simulink model "RW_Model"  (R2024a)
settings: Solver=VariableStepAuto  StartTime=0.0  StopTime=10.0  RelTol=1e-3
values from neighbouring files (symbols this model uses):
  b = 10e-6    (= 1e-05)    [init_SAR_AOCS.m]
  Km = 0.1    [init_SAR_AOCS.m]
  Kt = 0.1    [init_SAR_AOCS.m]
  L = 5.2e-3    (= 0.0052)    [init_SAR_AOCS.m]
  R = 2    [init_SAR_AOCS.m]
  rw_Inertia = 5e-4    (= 0.0005)    [init_SAR_AOCS.m]
  rw_SensorToBody = [0 0.4741 0.4741 -0.9482;                   -0.9999 0.3333 0.3333 0.3333;                    0 -0.8165 0.8165 0 ]    [init_SAR_AOCS.m]
  RW_wmax = 300    [init_SAR_AOCS.m]
  Ts = sim.dt    [init_SAR_AOCS.m]
  w_init = initial.omega    [init_SAR_AOCS.m]
  wRW_init = [0;0;0;0]    [init_SAR_AOCS.m]
libraries: simulink_extras x8, slpidlib x4, simulink x4
settings Model: Creator=hendr  LastModifiedBy=hendr

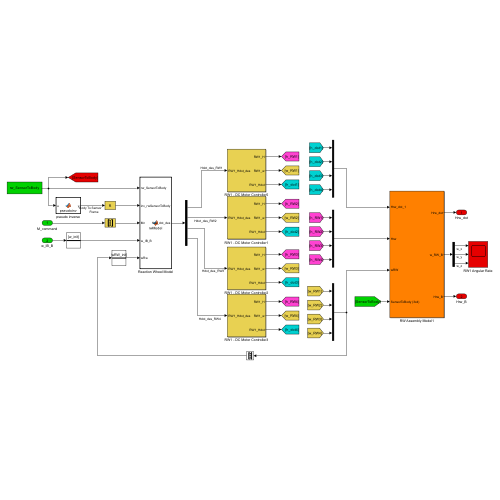
[thumbnail: Simulink's stored preview of the top-level diagram]
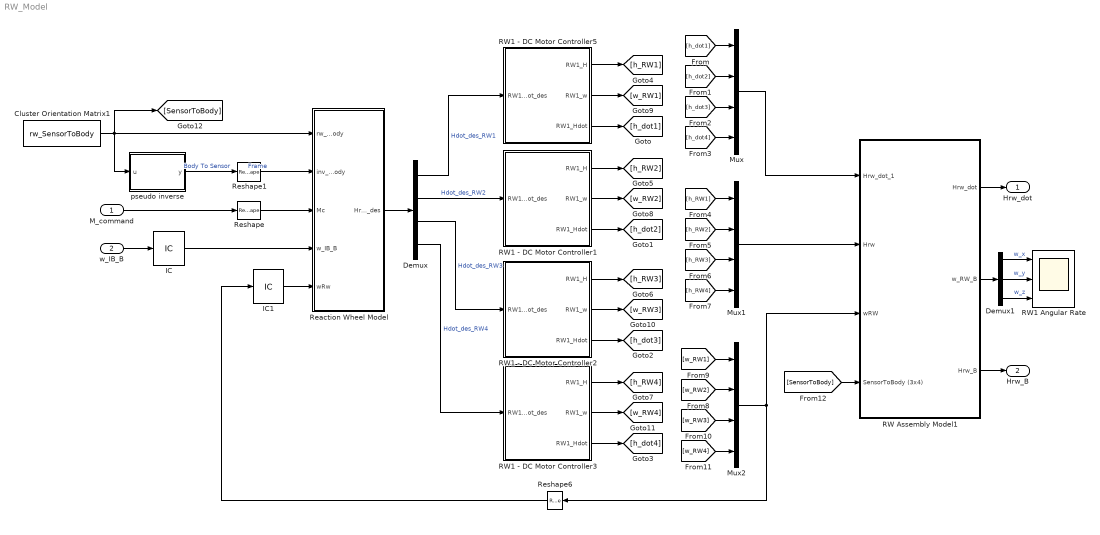
== system RW_Model ==
  "M_command " : Inport
  w_IB_B : Inport  Port=2
  Cluster Orientation Matrix1 : Constant  Value=rw_SensorToBody  VectorParams1D=off  SampleTime=Ts
  Demux : Demux
  Demux1 : Demux  Outputs=3
  IC : InitialCondition  Value=w_init
  IC1 : InitialCondition  Value=wRW_init
  Mux : Mux
  Mux1 : Mux
  Mux2 : Mux
  RW Assembly Model1 : Subsystem
  RW1 - DC Motor Controller1 : Subsystem
  RW1 - DC Motor Controller2 : Subsystem
  RW1 - DC Motor Controller3 : Subsystem
  RW1 - DC Motor Controller5 : Subsystem
  RW1 Angular Rate : Scope  NumInputPorts=3
  Reaction Wheel Model : MATLAB Function  TreatAsAtomicUnit=on
  Reshape : Reshape  OutputDimensionality=Column vector (2-D)
  Reshape1 : Reshape  OutputDimensionality=Customize  OutputDimensions=[4,3]
  Reshape6 : Reshape  OutputDimensionality=Column vector (2-D)
  pseudo inverse : MATLAB Function  TreatAsAtomicUnit=on
  "Hrw_dot " : Outport  VectorParamsAs1DForOutWhenUnconnected=off
  Hrw_B : Outport  Port=2  VectorParamsAs1DForOutWhenUnconnected=off
  wires:
  RW Assembly Model1/3(Hrw_B) -> Hrw_B/1
  Demux/4 -> RW1 - DC Motor Controller3/1(RW1_Hdot_des)  "Hdot_des_RW4"
  IC1/1 -> Reaction Wheel Model/5(wRw)
  Mux2/1 -> Reshape6/1, RW Assembly Model1/3(wRW)
  Reshape6/1 -> IC1/1
  RW1 - DC Motor Controller3/2(RW1_w) -> [w_RW4]
  RW1 - DC Motor Controller2/1(RW1_H) -> [h_RW3]
  RW1 - DC Motor Controller5/2(RW1_w) -> [w_RW1]
  [w_RW3] -> Mux2/3
  RW Assembly Model1/2(w_RW_B) -> Demux1/1
  RW1 - DC Motor Controller5/3(RW1_Hdot) -> [h_dot1]
  RW1 - DC Motor Controller3/3(RW1_Hdot) -> [h_dot4]
  RW1 - DC Motor Controller2/2(RW1_w) -> [w_RW3]
  RW1 - DC Motor Controller1/3(RW1_Hdot) -> [h_dot2]
  [h_dot3] -> Mux/3
  Demux/1 -> RW1 - DC Motor Controller5/1(RW1_Hdot_des)  "Hdot_des_RW1"
  RW1 - DC Motor Controller5/1(RW1_H) -> [h_RW1]
  RW1 - DC Motor Controller1/2(RW1_w) -> [w_RW2]
  RW1 - DC Motor Controller1/1(RW1_H) -> [h_RW2]
  RW1 - DC Motor Controller3/1(RW1_H) -> [h_RW4]
  RW1 - DC Motor Controller2/3(RW1_Hdot) -> [h_dot3]
  [h_RW3] -> Mux1/3
  Reshape1/1 -> Reaction Wheel Model/2(inv_rwSensorToBody)
  [SensorToBody] -> RW Assembly Model1/4(SensorToBody (3x4))
  "M_command "/1 -> Reshape/1
  Mux/1 -> RW Assembly Model1/1(Hrw_dot_1)
  Reshape/1 -> Reaction Wheel Model/3(Mc)
  pseudo inverse/1(y) -> Reshape1/1  "Body To Sensor         Frame"
  w_IB_B/1 -> IC/1
  Demux/2 -> RW1 - DC Motor Controller1/1(RW1_Hdot_des)  "Hdot_des_RW2"
  [h_RW2] -> Mux1/2
  RW Assembly Model1/1(Hrw_dot) -> "Hrw_dot "/1
  IC/1 -> Reaction Wheel Model/4(w_IB_B)
  [h_RW4] -> Mux1/4
  Demux1/3 -> RW1 Angular Rate/3  "w_z"
  [w_RW2] -> Mux2/2
  [h_RW1] -> Mux1/1
  [h_dot2] -> Mux/2
  Reaction Wheel Model/1(Hrw_dot_des) -> Demux/1
  [w_RW1] -> Mux2/1
  Demux/3 -> RW1 - DC Motor Controller2/1(RW1_Hdot_des)  "Hdot_des_RW3"
  Mux1/1 -> RW Assembly Model1/2(Hrw)
  [h_dot4] -> Mux/4
  [w_RW4] -> Mux2/4
  Cluster Orientation Matrix1/1 -> pseudo inverse/1(u), [SensorToBody], Reaction Wheel Model/1(rw_SensorToBody)
  Demux1/1 -> RW1 Angular Rate/1  "w_x"
  [h_dot1] -> Mux/1
  Demux1/2 -> RW1 Angular Rate/2  "w_y"

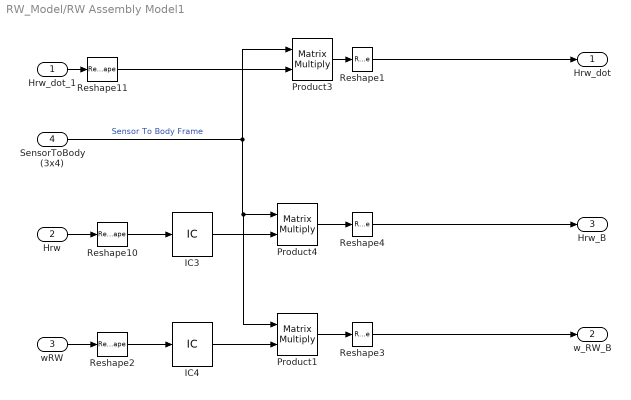
== system RW_Model/RW Assembly Model1 ==
  Hrw_dot_1 : Inport
  Hrw : Inport  Port=2
  wRW : Inport  Port=3
  SensorToBody (3x4) : Inport  Port=4
  IC3 : InitialCondition  Value=[wRW_init(1,1)*rw_Inertia; wRW_init(2,1)*rw_Inertia; wRW_init(3,1)*rw_Inertia;wRW_init(4,1)*rw_Inertia]
  IC4 : InitialCondition  Value=wRW_init
  Product1 : Product  Inputs=**  Multiplication=Matrix(*)  RndMeth=Zero
  Product3 : Product  Inputs=**  Multiplication=Matrix(*)  RndMeth=Zero
  Product4 : Product  Inputs=**  Multiplication=Matrix(*)  RndMeth=Zero
  Reshape{1..4,10..11} (6 alike) : Reshape  OutputDimensionality=Column vector (2-D)
  Hrw_dot : Outport  VectorParamsAs1DForOutWhenUnconnected=off
  w_RW_B : Outport  Port=2  VectorParamsAs1DForOutWhenUnconnected=off
  Hrw_B : Outport  Port=3  VectorParamsAs1DForOutWhenUnconnected=off
  wires:
  SensorToBody (3x4)/1 -> Product3/1, Product1/1, Product4/1  "Sensor To Body Frame"
  Product4/1 -> Reshape4/1
  Reshape1/1 -> Hrw_dot/1
  Reshape4/1 -> Hrw_B/1
  IC3/1 -> Product4/2
  IC4/1 -> Product1/2
  Product1/1 -> Reshape3/1
  Hrw/1 -> Reshape10/1
  Reshape10/1 -> IC3/1
  Reshape2/1 -> IC4/1
  wRW/1 -> Reshape2/1
  Reshape3/1 -> w_RW_B/1
  Reshape11/1 -> Product3/2
  Hrw_dot_1/1 -> Reshape11/1
  Product3/1 -> Reshape1/1

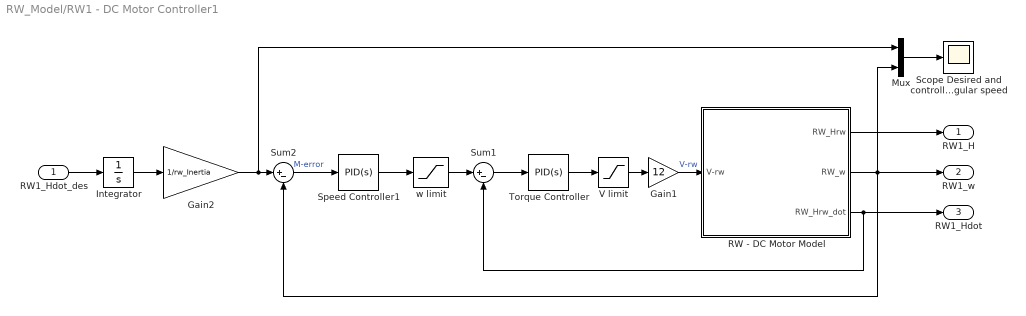
== system RW_Model/RW1 - DC Motor Controller1 ==
  RW1_Hdot_des : Inport
  Gain1 : Gain  Gain=12
  Gain2 : Gain  Gain=1/rw_Inertia
  Integrator : Integrator
  Mux : Mux  Inputs=2
  RW - DC Motor Model : Subsystem
  "Scope Desired and controlled RW-angular speed " : Scope
  Speed Controller1 : slpidlib/PID Controller  Controller=PID  Form=Parallel  TimeDomain=Continuous-time  UseExternalTs=off  SampleTime=0.01  IntegratorMethod=Forward Euler  FilterMethod=Forward Euler  ControllerParametersSource=internal  P=9.56052273582853  I=13.4366327144231  UseKiTs=off  D=1.16248121318414  UseExternalDerivativeSource=off  N=2668.95305381072  UseFilter=on  TunerSelectOption=Transfer Function Based (PID Tuner App)  InitialConditionSource=internal  InitialConditionForIntegrator=0  InitialConditionForFilter=0  DifferentiatorICPrevScaledInput=0  ExternalReset=none  TrackingMode=off  Kt=1  LimitOutput=off  SatLimitsSource=internal  UpperSaturationLimit=inf  LowerSaturationLimit=-inf  LinearizeAsGain=on  AntiWindupMode=none  Kb=1  LimitIntegrator=off  UpperIntegratorSaturationLimit=inf  LowerIntegratorSaturationLimit=-inf  POutMin=[]  POutMax=[]  IOutMin=[]  IOutMax=[]  DOutMin=[]  DOutMax=[]  NOutMin=[]  NOutMax=[]  SumOutMin=[]  SumOutMax=[]  SaturationOutMin=[]  SaturationOutMax=[]  PParamMin=[]  PParamMax=[]  IParamMin=[]  IParamMax=[]  DParamMin=[]  DParamMax=[]  NParamMin=[]  NParamMax=[]  KbParamMin=[]  KbParamMax=[]  KtParamMin=[]  KtParamMax=[]  KbOutMin=[]  KbOutMax=[]  KtOutMin=[]  KtOutMax=[]  IntegratorOutMin=[]  IntegratorOutMax=[]  FilterOutMin=[]  FilterOutMax=[]  SumI1OutMin=[]  SumI1OutMax=[]  SumI2OutMin=[]  SumI2OutMax=[]  SumI3OutMin=[]  SumI3OutMax=[]  SumI4OutMin=[]  SumI4OutMax=[]  SumDOutMin=[]  SumDOutMax=[]  DifferentiatorOutMin=[]  DifferentiatorOutMax=[]  FilterDiffOutCoefMin=[]  FilterDiffOutCoefMax=[]  ReciprocalOutMin=[]  ReciprocalOutMax=[]  SumDenOutMin=[]  SumDenOutMax=[]  SumNumOutMin=[]  SumNumOutMax=[]  DivideOutMin=[]  DivideOutMax=[]  UdiffTsProdOutMin=[]  UdiffTsProdOutMax=[]  NTsProdOutMin=[]  NTsProdOutMax=[]  UintegralTsProdOutMin=[]  UintegralTsProdOutMax=[]  UngainTsProdOutMin=[]  UngainTsProdOutMax=[]  ClampingZeroOutDataTypeStr=Inherit: Inherit via back propagation  ClampingZeroOutMin=[]  ClampingZeroOutMax=[]  FilterDenConstantOutDataTypeStr=Inherit: Inherit via back propagation  FilterDenConstantOutMin=[]  FilterDenConstantOutMax=[]  PCopyOutDataTypeStr=Inherit: Inherit via back propagation  PCopyOutMin=[]  PCopyOutMax=[]  NCopyOutDataTypeStr=Inherit: Inherit via back propagation  NCopyOutMin=[]  NCopyOutMax=[]  IntegratorContinuousStateAttributes=''  IntegratorStateMustResolveToSignalObject=off  IntegratorRTWStateStorageClass=Auto  FilterContinuousStateAttributes=''  FilterStateMustResolveToSignalObject=off  FilterRTWStateStorageClass=Auto  ParallelPVariant=InternalParameters  IdealPVariant=Disabled  IVariant=InternalParameters  DVariant=InternalParameters  IntegratorVariant=Continuous  SatVariant=Disabled  AWVariant=Passthrough  PCopyVariant=Disabled  TRVariant=Disabled  FdbkBlocksVariant=Forward  IdealPFdbkVariant=Disabled  SatFdbkVariant=Disabled  DerivativeFilterVariant=ContFilter  NVariant=InternalParameters  NCopyVariant=Disabled  FilterICVariant=InternalICsFilter  IntegratorICVariant=InternalICs  ExternalResetVariant=Disabled  TRSumVariant=Passthrough  SumFdbkVariant=Disabled  SumVariant=Sum_PID  TsampFilterVariant=InternalTs  TsampNgainVariant=Passthrough  TsampIntegralVariant=Disabled_SignalSpec  ExternalSaturationOutDataTypeStr=Inherit: Same as second input  DerivativeSourceVariant=ErrorSignal
  Sum1 : Sum  Inputs=|+-
  Sum2 : Sum  Inputs=|+-
  Torque Controller : slpidlib/PID Controller  Controller=PID  Form=Parallel  TimeDomain=Continuous-time  UseExternalTs=off  SampleTime=0.01  IntegratorMethod=Forward Euler  FilterMethod=Forward Euler  ControllerParametersSource=internal  P=2.50374683332827e-05  I=0.022215359014968  UseKiTs=off  D=0  UseExternalDerivativeSource=off  N=100  UseFilter=on  TunerSelectOption=Transfer Function Based (PID Tuner App)  InitialConditionSource=internal  InitialConditionForIntegrator=0  InitialConditionForFilter=0  DifferentiatorICPrevScaledInput=0  ExternalReset=none  TrackingMode=off  Kt=1  LimitOutput=off  SatLimitsSource=internal  UpperSaturationLimit=inf  LowerSaturationLimit=-inf  LinearizeAsGain=on  AntiWindupMode=none  Kb=1  LimitIntegrator=off  UpperIntegratorSaturationLimit=inf  LowerIntegratorSaturationLimit=-inf  POutMin=[]  POutMax=[]  IOutMin=[]  IOutMax=[]  DOutMin=[]  DOutMax=[]  NOutMin=[]  NOutMax=[]  SumOutMin=[]  SumOutMax=[]  SaturationOutMin=[]  SaturationOutMax=[]  PParamMin=[]  PParamMax=[]  IParamMin=[]  IParamMax=[]  DParamMin=[]  DParamMax=[]  NParamMin=[]  NParamMax=[]  KbParamMin=[]  KbParamMax=[]  KtParamMin=[]  KtParamMax=[]  KbOutMin=[]  KbOutMax=[]  KtOutMin=[]  KtOutMax=[]  IntegratorOutMin=[]  IntegratorOutMax=[]  FilterOutMin=[]  FilterOutMax=[]  SumI1OutMin=[]  SumI1OutMax=[]  SumI2OutMin=[]  SumI2OutMax=[]  SumI3OutMin=[]  SumI3OutMax=[]  SumI4OutMin=[]  SumI4OutMax=[]  SumDOutMin=[]  SumDOutMax=[]  DifferentiatorOutMin=[]  DifferentiatorOutMax=[]  FilterDiffOutCoefMin=[]  FilterDiffOutCoefMax=[]  ReciprocalOutMin=[]  ReciprocalOutMax=[]  SumDenOutMin=[]  SumDenOutMax=[]  SumNumOutMin=[]  SumNumOutMax=[]  DivideOutMin=[]  DivideOutMax=[]  UdiffTsProdOutMin=[]  UdiffTsProdOutMax=[]  NTsProdOutMin=[]  NTsProdOutMax=[]  UintegralTsProdOutMin=[]  UintegralTsProdOutMax=[]  UngainTsProdOutMin=[]  UngainTsProdOutMax=[]  ClampingZeroOutDataTypeStr=Inherit: Inherit via back propagation  ClampingZeroOutMin=[]  ClampingZeroOutMax=[]  FilterDenConstantOutDataTypeStr=Inherit: Inherit via back propagation  FilterDenConstantOutMin=[]  FilterDenConstantOutMax=[]  PCopyOutDataTypeStr=Inherit: Inherit via back propagation  PCopyOutMin=[]  PCopyOutMax=[]  NCopyOutDataTypeStr=Inherit: Inherit via back propagation  NCopyOutMin=[]  NCopyOutMax=[]  IntegratorContinuousStateAttributes=''  IntegratorStateMustResolveToSignalObject=off  IntegratorRTWStateStorageClass=Auto  FilterContinuousStateAttributes=''  FilterStateMustResolveToSignalObject=off  FilterRTWStateStorageClass=Auto  ParallelPVariant=InternalParameters  IdealPVariant=Disabled  IVariant=InternalParameters  DVariant=InternalParameters  IntegratorVariant=Continuous  SatVariant=Disabled  AWVariant=Passthrough  PCopyVariant=Disabled  TRVariant=Disabled  FdbkBlocksVariant=Forward  IdealPFdbkVariant=Disabled  SatFdbkVariant=Disabled  DerivativeFilterVariant=ContFilter  NVariant=InternalParameters  NCopyVariant=Disabled  FilterICVariant=InternalICsFilter  IntegratorICVariant=InternalICs  ExternalResetVariant=Disabled  TRSumVariant=Passthrough  SumFdbkVariant=Disabled  SumVariant=Sum_PID  TsampFilterVariant=InternalTs  TsampNgainVariant=Passthrough  TsampIntegralVariant=Disabled_SignalSpec  ExternalSaturationOutDataTypeStr=Inherit: Same as second input  DerivativeSourceVariant=ErrorSignal
  V limit : Saturate  UpperLimit=20  LowerLimit=-20
  w limit : Saturate  UpperLimit=RW_wmax  LowerLimit=-RW_wmax
  RW1_H : Outport  VectorParamsAs1DForOutWhenUnconnected=off
  RW1_w : Outport  Port=2  VectorParamsAs1DForOutWhenUnconnected=off
  RW1_Hdot : Outport  Port=3  VectorParamsAs1DForOutWhenUnconnected=off
  wires:
  Torque Controller/1 -> V limit/1
  RW - DC Motor Model/3(RW_Hrw_dot) -> RW1_Hdot/1, Sum1/2
  Mux/1 -> "Scope Desired and controlled RW-angular speed "/1
  V limit/1 -> Gain1/1
  Gain1/1 -> RW - DC Motor Model/1(V-rw)  "V-rw"
  RW - DC Motor Model/2(RW_w) -> RW1_w/1, Sum2/2, Mux/2
  Sum1/1 -> Torque Controller/1
  RW - DC Motor Model/1(RW_Hrw) -> RW1_H/1
  Speed Controller1/1 -> w limit/1
  w limit/1 -> Sum1/1
  Sum2/1 -> Speed Controller1/1  "M-error"
  Integrator/1 -> Gain2/1
  RW1_Hdot_des/1 -> Integrator/1
  Gain2/1 -> Mux/1, Sum2/1

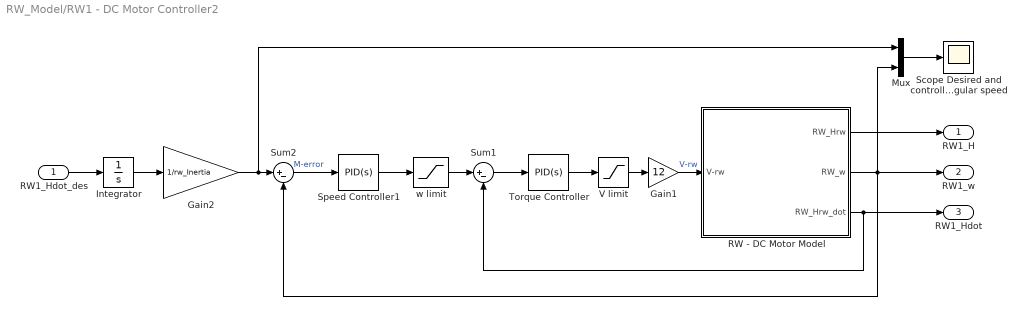
== system RW_Model/RW1 - DC Motor Controller2 ==
  RW1_Hdot_des : Inport
  Gain1 : Gain  Gain=12
  Gain2 : Gain  Gain=1/rw_Inertia
  Integrator : Integrator
  Mux : Mux  Inputs=2
  RW - DC Motor Model : Subsystem
  "Scope Desired and controlled RW-angular speed " : Scope
  Speed Controller1 : simulink/Continuous/PID Controller  Controller=PID  Form=Parallel  TimeDomain=Continuous-time  SampleTime=0.01  IntegratorMethod=Forward Euler  FilterMethod=Forward Euler  ControllerParametersSource=internal  P=9.56052273582853  I=13.4366327144231  D=1.16248121318414  UseFilter=on  N=2668.95305381072  TunerSelectOption=Transfer Function Based (PID Tuner App)  InitialConditionSource=internal  InitialConditionForIntegrator=0  InitialConditionForFilter=0  DifferentiatorICPrevScaledInput=0  ExternalReset=none  TrackingMode=off  Kt=1  LimitOutput=off  UpperSaturationLimit=inf  LowerSaturationLimit=-inf  LinearizeAsGain=on  AntiWindupMode=none  Kb=1  POutMin=[]  POutMax=[]  IOutMin=[]  IOutMax=[]  DOutMin=[]  DOutMax=[]  NOutMin=[]  NOutMax=[]  SumOutMin=[]  SumOutMax=[]  SaturationOutMin=[]  SaturationOutMax=[]  PParamMin=[]  PParamMax=[]  IParamMin=[]  IParamMax=[]  DParamMin=[]  DParamMax=[]  NParamMin=[]  NParamMax=[]  KbParamMin=[]  KbParamMax=[]  KtParamMin=[]  KtParamMax=[]  KbOutMin=[]  KbOutMax=[]  KtOutMin=[]  KtOutMax=[]  IntegratorOutMin=[]  IntegratorOutMax=[]  FilterOutMin=[]  FilterOutMax=[]  SumI1OutMin=[]  SumI1OutMax=[]  SumI2OutMin=[]  SumI2OutMax=[]  SumI3OutMin=[]  SumI3OutMax=[]  SumI4OutMin=[]  SumI4OutMax=[]  SumDOutMin=[]  SumDOutMax=[]  DifferentiatorOutMin=[]  DifferentiatorOutMax=[]  FilterDiffOutCoefMin=[]  FilterDiffOutCoefMax=[]  ReciprocalOutMin=[]  ReciprocalOutMax=[]  SumDenOutMin=[]  SumDenOutMax=[]  SumNumOutMin=[]  SumNumOutMax=[]  DivideOutMin=[]  DivideOutMax=[]  IntegratorContinuousStateAttributes=''  IntegratorStateMustResolveToSignalObject=off  IntegratorRTWStateStorageClass=Auto  FilterContinuousStateAttributes=''  FilterStateMustResolveToSignalObject=off  FilterRTWStateStorageClass=Auto  ParallelPVariant=InternalParameters  IdealPVariant=Disabled  IVariant=InternalParameters  DVariant=InternalParameters  IntegratorVariant=Continuous  SatVariant=Disabled  AWVariant=Passthrough  PCopyVariant=Disabled  TRVariant=Disabled  FdbkBlocksVariant=Forward  IdealPFdbkVariant=Disabled  SatFdbkVariant=Disabled  DerivativeFilterVariant=ContFilter  NVariant=InternalParameters  NCopyVariant=Disabled  FilterICVariant=InternalICsFilter  IntegratorICVariant=InternalICs  ExternalResetVariant=Disabled  TRSumVariant=Passthrough  SumFdbkVariant=Disabled  SumVariant=Sum_PID
  Sum1 : Sum  Inputs=|+-
  Sum2 : Sum  Inputs=|+-
  Torque Controller : simulink/Continuous/PID Controller  Controller=PID  Form=Parallel  TimeDomain=Continuous-time  SampleTime=0.01  IntegratorMethod=Forward Euler  FilterMethod=Forward Euler  ControllerParametersSource=internal  P=2.50374683332827e-05  I=0.022215359014968  D=0  UseFilter=on  N=100  TunerSelectOption=Transfer Function Based (PID Tuner App)  InitialConditionSource=internal  InitialConditionForIntegrator=0  InitialConditionForFilter=0  DifferentiatorICPrevScaledInput=0  ExternalReset=none  TrackingMode=off  Kt=1  LimitOutput=off  UpperSaturationLimit=inf  LowerSaturationLimit=-inf  LinearizeAsGain=on  AntiWindupMode=none  Kb=1  POutMin=[]  POutMax=[]  IOutMin=[]  IOutMax=[]  DOutMin=[]  DOutMax=[]  NOutMin=[]  NOutMax=[]  SumOutMin=[]  SumOutMax=[]  SaturationOutMin=[]  SaturationOutMax=[]  PParamMin=[]  PParamMax=[]  IParamMin=[]  IParamMax=[]  DParamMin=[]  DParamMax=[]  NParamMin=[]  NParamMax=[]  KbParamMin=[]  KbParamMax=[]  KtParamMin=[]  KtParamMax=[]  KbOutMin=[]  KbOutMax=[]  KtOutMin=[]  KtOutMax=[]  IntegratorOutMin=[]  IntegratorOutMax=[]  FilterOutMin=[]  FilterOutMax=[]  SumI1OutMin=[]  SumI1OutMax=[]  SumI2OutMin=[]  SumI2OutMax=[]  SumI3OutMin=[]  SumI3OutMax=[]  SumI4OutMin=[]  SumI4OutMax=[]  SumDOutMin=[]  SumDOutMax=[]  DifferentiatorOutMin=[]  DifferentiatorOutMax=[]  FilterDiffOutCoefMin=[]  FilterDiffOutCoefMax=[]  ReciprocalOutMin=[]  ReciprocalOutMax=[]  SumDenOutMin=[]  SumDenOutMax=[]  SumNumOutMin=[]  SumNumOutMax=[]  DivideOutMin=[]  DivideOutMax=[]  IntegratorContinuousStateAttributes=''  IntegratorStateMustResolveToSignalObject=off  IntegratorRTWStateStorageClass=Auto  FilterContinuousStateAttributes=''  FilterStateMustResolveToSignalObject=off  FilterRTWStateStorageClass=Auto  ParallelPVariant=InternalParameters  IdealPVariant=Disabled  IVariant=InternalParameters  DVariant=InternalParameters  IntegratorVariant=Continuous  SatVariant=Disabled  AWVariant=Passthrough  PCopyVariant=Disabled  TRVariant=Disabled  FdbkBlocksVariant=Forward  IdealPFdbkVariant=Disabled  SatFdbkVariant=Disabled  DerivativeFilterVariant=ContFilter  NVariant=InternalParameters  NCopyVariant=Disabled  FilterICVariant=InternalICsFilter  IntegratorICVariant=InternalICs  ExternalResetVariant=Disabled  TRSumVariant=Passthrough  SumFdbkVariant=Disabled  SumVariant=Sum_PID
  V limit : Saturate  UpperLimit=20  LowerLimit=-20
  w limit : Saturate  UpperLimit=RW_wmax  LowerLimit=-RW_wmax
  RW1_H : Outport  VectorParamsAs1DForOutWhenUnconnected=off
  RW1_w : Outport  Port=2  VectorParamsAs1DForOutWhenUnconnected=off
  RW1_Hdot : Outport  Port=3  VectorParamsAs1DForOutWhenUnconnected=off
  wires:
  Torque Controller/1 -> V limit/1
  RW - DC Motor Model/3(RW_Hrw_dot) -> RW1_Hdot/1, Sum1/2
  Mux/1 -> "Scope Desired and controlled RW-angular speed "/1
  V limit/1 -> Gain1/1
  Gain1/1 -> RW - DC Motor Model/1(V-rw)  "V-rw"
  RW - DC Motor Model/2(RW_w) -> RW1_w/1, Sum2/2, Mux/2
  Sum1/1 -> Torque Controller/1
  RW - DC Motor Model/1(RW_Hrw) -> RW1_H/1
  Speed Controller1/1 -> w limit/1
  w limit/1 -> Sum1/1
  Sum2/1 -> Speed Controller1/1  "M-error"
  Integrator/1 -> Gain2/1
  RW1_Hdot_des/1 -> Integrator/1
  Gain2/1 -> Mux/1, Sum2/1

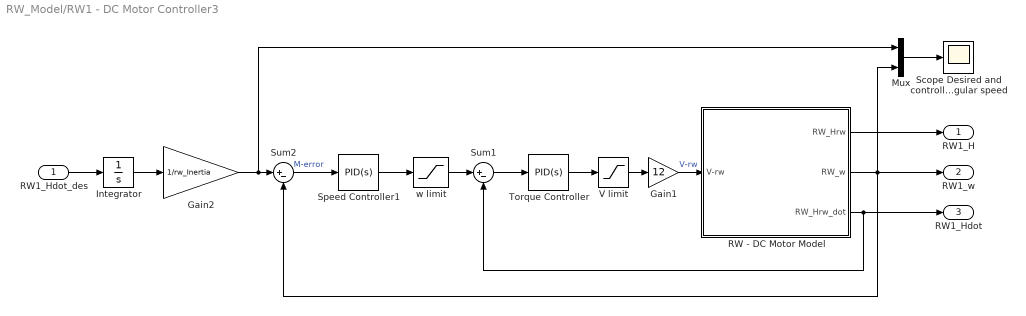
== system RW_Model/RW1 - DC Motor Controller3 ==
  RW1_Hdot_des : Inport
  Gain1 : Gain  Gain=12
  Gain2 : Gain  Gain=1/rw_Inertia
  Integrator : Integrator
  Mux : Mux  Inputs=2
  RW - DC Motor Model : Subsystem
  "Scope Desired and controlled RW-angular speed " : Scope
  Speed Controller1 : simulink/Continuous/PID Controller  Controller=PID  Form=Parallel  TimeDomain=Continuous-time  SampleTime=0.01  IntegratorMethod=Forward Euler  FilterMethod=Forward Euler  ControllerParametersSource=internal  P=9.56052273582853  I=13.4366327144231  D=1.16248121318414  UseFilter=on  N=2668.95305381072  TunerSelectOption=Transfer Function Based (PID Tuner App)  InitialConditionSource=internal  InitialConditionForIntegrator=0  InitialConditionForFilter=0  DifferentiatorICPrevScaledInput=0  ExternalReset=none  TrackingMode=off  Kt=1  LimitOutput=off  UpperSaturationLimit=inf  LowerSaturationLimit=-inf  LinearizeAsGain=on  AntiWindupMode=none  Kb=1  POutMin=[]  POutMax=[]  IOutMin=[]  IOutMax=[]  DOutMin=[]  DOutMax=[]  NOutMin=[]  NOutMax=[]  SumOutMin=[]  SumOutMax=[]  SaturationOutMin=[]  SaturationOutMax=[]  PParamMin=[]  PParamMax=[]  IParamMin=[]  IParamMax=[]  DParamMin=[]  DParamMax=[]  NParamMin=[]  NParamMax=[]  KbParamMin=[]  KbParamMax=[]  KtParamMin=[]  KtParamMax=[]  KbOutMin=[]  KbOutMax=[]  KtOutMin=[]  KtOutMax=[]  IntegratorOutMin=[]  IntegratorOutMax=[]  FilterOutMin=[]  FilterOutMax=[]  SumI1OutMin=[]  SumI1OutMax=[]  SumI2OutMin=[]  SumI2OutMax=[]  SumI3OutMin=[]  SumI3OutMax=[]  SumI4OutMin=[]  SumI4OutMax=[]  SumDOutMin=[]  SumDOutMax=[]  DifferentiatorOutMin=[]  DifferentiatorOutMax=[]  FilterDiffOutCoefMin=[]  FilterDiffOutCoefMax=[]  ReciprocalOutMin=[]  ReciprocalOutMax=[]  SumDenOutMin=[]  SumDenOutMax=[]  SumNumOutMin=[]  SumNumOutMax=[]  DivideOutMin=[]  DivideOutMax=[]  IntegratorContinuousStateAttributes=''  IntegratorStateMustResolveToSignalObject=off  IntegratorRTWStateStorageClass=Auto  FilterContinuousStateAttributes=''  FilterStateMustResolveToSignalObject=off  FilterRTWStateStorageClass=Auto  ParallelPVariant=InternalParameters  IdealPVariant=Disabled  IVariant=InternalParameters  DVariant=InternalParameters  IntegratorVariant=Continuous  SatVariant=Disabled  AWVariant=Passthrough  PCopyVariant=Disabled  TRVariant=Disabled  FdbkBlocksVariant=Forward  IdealPFdbkVariant=Disabled  SatFdbkVariant=Disabled  DerivativeFilterVariant=ContFilter  NVariant=InternalParameters  NCopyVariant=Disabled  FilterICVariant=InternalICsFilter  IntegratorICVariant=InternalICs  ExternalResetVariant=Disabled  TRSumVariant=Passthrough  SumFdbkVariant=Disabled  SumVariant=Sum_PID
  Sum1 : Sum  Inputs=|+-
  Sum2 : Sum  Inputs=|+-
  Torque Controller : simulink/Continuous/PID Controller  Controller=PID  Form=Parallel  TimeDomain=Continuous-time  SampleTime=0.01  IntegratorMethod=Forward Euler  FilterMethod=Forward Euler  ControllerParametersSource=internal  P=2.50374683332827e-05  I=0.022215359014968  D=0  UseFilter=on  N=100  TunerSelectOption=Transfer Function Based (PID Tuner App)  InitialConditionSource=internal  InitialConditionForIntegrator=0  InitialConditionForFilter=0  DifferentiatorICPrevScaledInput=0  ExternalReset=none  TrackingMode=off  Kt=1  LimitOutput=off  UpperSaturationLimit=inf  LowerSaturationLimit=-inf  LinearizeAsGain=on  AntiWindupMode=none  Kb=1  POutMin=[]  POutMax=[]  IOutMin=[]  IOutMax=[]  DOutMin=[]  DOutMax=[]  NOutMin=[]  NOutMax=[]  SumOutMin=[]  SumOutMax=[]  SaturationOutMin=[]  SaturationOutMax=[]  PParamMin=[]  PParamMax=[]  IParamMin=[]  IParamMax=[]  DParamMin=[]  DParamMax=[]  NParamMin=[]  NParamMax=[]  KbParamMin=[]  KbParamMax=[]  KtParamMin=[]  KtParamMax=[]  KbOutMin=[]  KbOutMax=[]  KtOutMin=[]  KtOutMax=[]  IntegratorOutMin=[]  IntegratorOutMax=[]  FilterOutMin=[]  FilterOutMax=[]  SumI1OutMin=[]  SumI1OutMax=[]  SumI2OutMin=[]  SumI2OutMax=[]  SumI3OutMin=[]  SumI3OutMax=[]  SumI4OutMin=[]  SumI4OutMax=[]  SumDOutMin=[]  SumDOutMax=[]  DifferentiatorOutMin=[]  DifferentiatorOutMax=[]  FilterDiffOutCoefMin=[]  FilterDiffOutCoefMax=[]  ReciprocalOutMin=[]  ReciprocalOutMax=[]  SumDenOutMin=[]  SumDenOutMax=[]  SumNumOutMin=[]  SumNumOutMax=[]  DivideOutMin=[]  DivideOutMax=[]  IntegratorContinuousStateAttributes=''  IntegratorStateMustResolveToSignalObject=off  IntegratorRTWStateStorageClass=Auto  FilterContinuousStateAttributes=''  FilterStateMustResolveToSignalObject=off  FilterRTWStateStorageClass=Auto  ParallelPVariant=InternalParameters  IdealPVariant=Disabled  IVariant=InternalParameters  DVariant=InternalParameters  IntegratorVariant=Continuous  SatVariant=Disabled  AWVariant=Passthrough  PCopyVariant=Disabled  TRVariant=Disabled  FdbkBlocksVariant=Forward  IdealPFdbkVariant=Disabled  SatFdbkVariant=Disabled  DerivativeFilterVariant=ContFilter  NVariant=InternalParameters  NCopyVariant=Disabled  FilterICVariant=InternalICsFilter  IntegratorICVariant=InternalICs  ExternalResetVariant=Disabled  TRSumVariant=Passthrough  SumFdbkVariant=Disabled  SumVariant=Sum_PID
  V limit : Saturate  UpperLimit=20  LowerLimit=-20
  w limit : Saturate  UpperLimit=RW_wmax  LowerLimit=-RW_wmax
  RW1_H : Outport  VectorParamsAs1DForOutWhenUnconnected=off
  RW1_w : Outport  Port=2  VectorParamsAs1DForOutWhenUnconnected=off
  RW1_Hdot : Outport  Port=3  VectorParamsAs1DForOutWhenUnconnected=off
  wires:
  Torque Controller/1 -> V limit/1
  RW - DC Motor Model/3(RW_Hrw_dot) -> RW1_Hdot/1, Sum1/2
  Mux/1 -> "Scope Desired and controlled RW-angular speed "/1
  V limit/1 -> Gain1/1
  Gain1/1 -> RW - DC Motor Model/1(V-rw)  "V-rw"
  RW - DC Motor Model/2(RW_w) -> RW1_w/1, Sum2/2, Mux/2
  Sum1/1 -> Torque Controller/1
  RW - DC Motor Model/1(RW_Hrw) -> RW1_H/1
  Speed Controller1/1 -> w limit/1
  w limit/1 -> Sum1/1
  Sum2/1 -> Speed Controller1/1  "M-error"
  Integrator/1 -> Gain2/1
  RW1_Hdot_des/1 -> Integrator/1
  Gain2/1 -> Mux/1, Sum2/1

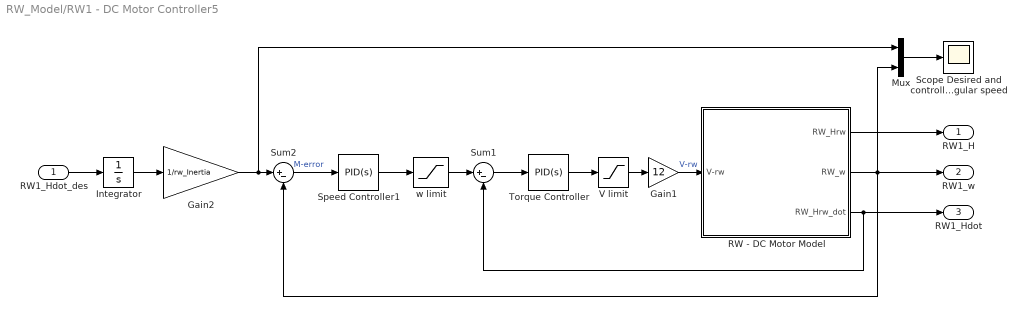
== system RW_Model/RW1 - DC Motor Controller5 ==
  RW1_Hdot_des : Inport
  Gain1 : Gain  Gain=12
  Gain2 : Gain  Gain=1/rw_Inertia
  Integrator : Integrator
  Mux : Mux  Inputs=2
  RW - DC Motor Model : Subsystem
  "Scope Desired and controlled RW-angular speed " : Scope
  Speed Controller1 : slpidlib/PID Controller  Controller=PID  Form=Parallel  TimeDomain=Continuous-time  UseExternalTs=off  SampleTime=0.01  IntegratorMethod=Forward Euler  FilterMethod=Forward Euler  ControllerParametersSource=internal  P=9.56052273582853  I=13.4366327144231  UseKiTs=off  D=1.16248121318414  UseExternalDerivativeSource=off  N=2668.95305381072  UseFilter=on  TunerSelectOption=Transfer Function Based (PID Tuner App)  InitialConditionSource=internal  InitialConditionForIntegrator=0  InitialConditionForFilter=0  DifferentiatorICPrevScaledInput=0  ExternalReset=none  TrackingMode=off  Kt=1  LimitOutput=off  SatLimitsSource=internal  UpperSaturationLimit=inf  LowerSaturationLimit=-inf  LinearizeAsGain=on  AntiWindupMode=none  Kb=1  LimitIntegrator=off  UpperIntegratorSaturationLimit=inf  LowerIntegratorSaturationLimit=-inf  POutMin=[]  POutMax=[]  IOutMin=[]  IOutMax=[]  DOutMin=[]  DOutMax=[]  NOutMin=[]  NOutMax=[]  SumOutMin=[]  SumOutMax=[]  SaturationOutMin=[]  SaturationOutMax=[]  PParamMin=[]  PParamMax=[]  IParamMin=[]  IParamMax=[]  DParamMin=[]  DParamMax=[]  NParamMin=[]  NParamMax=[]  KbParamMin=[]  KbParamMax=[]  KtParamMin=[]  KtParamMax=[]  KbOutMin=[]  KbOutMax=[]  KtOutMin=[]  KtOutMax=[]  IntegratorOutMin=[]  IntegratorOutMax=[]  FilterOutMin=[]  FilterOutMax=[]  SumI1OutMin=[]  SumI1OutMax=[]  SumI2OutMin=[]  SumI2OutMax=[]  SumI3OutMin=[]  SumI3OutMax=[]  SumI4OutMin=[]  SumI4OutMax=[]  SumDOutMin=[]  SumDOutMax=[]  DifferentiatorOutMin=[]  DifferentiatorOutMax=[]  FilterDiffOutCoefMin=[]  FilterDiffOutCoefMax=[]  ReciprocalOutMin=[]  ReciprocalOutMax=[]  SumDenOutMin=[]  SumDenOutMax=[]  SumNumOutMin=[]  SumNumOutMax=[]  DivideOutMin=[]  DivideOutMax=[]  UdiffTsProdOutMin=[]  UdiffTsProdOutMax=[]  NTsProdOutMin=[]  NTsProdOutMax=[]  UintegralTsProdOutMin=[]  UintegralTsProdOutMax=[]  UngainTsProdOutMin=[]  UngainTsProdOutMax=[]  ClampingZeroOutDataTypeStr=Inherit: Inherit via back propagation  ClampingZeroOutMin=[]  ClampingZeroOutMax=[]  FilterDenConstantOutDataTypeStr=Inherit: Inherit via back propagation  FilterDenConstantOutMin=[]  FilterDenConstantOutMax=[]  PCopyOutDataTypeStr=Inherit: Inherit via back propagation  PCopyOutMin=[]  PCopyOutMax=[]  NCopyOutDataTypeStr=Inherit: Inherit via back propagation  NCopyOutMin=[]  NCopyOutMax=[]  IntegratorContinuousStateAttributes=''  IntegratorStateMustResolveToSignalObject=off  IntegratorRTWStateStorageClass=Auto  FilterContinuousStateAttributes=''  FilterStateMustResolveToSignalObject=off  FilterRTWStateStorageClass=Auto  ParallelPVariant=InternalParameters  IdealPVariant=Disabled  IVariant=InternalParameters  DVariant=InternalParameters  IntegratorVariant=Continuous  SatVariant=Disabled  AWVariant=Passthrough  PCopyVariant=Disabled  TRVariant=Disabled  FdbkBlocksVariant=Forward  IdealPFdbkVariant=Disabled  SatFdbkVariant=Disabled  DerivativeFilterVariant=ContFilter  NVariant=InternalParameters  NCopyVariant=Disabled  FilterICVariant=InternalICsFilter  IntegratorICVariant=InternalICs  ExternalResetVariant=Disabled  TRSumVariant=Passthrough  SumFdbkVariant=Disabled  SumVariant=Sum_PID  TsampFilterVariant=InternalTs  TsampNgainVariant=Passthrough  TsampIntegralVariant=Disabled_SignalSpec  ExternalSaturationOutDataTypeStr=Inherit: Same as second input  DerivativeSourceVariant=ErrorSignal
  Sum1 : Sum  Inputs=|+-
  Sum2 : Sum  Inputs=|+-
  Torque Controller : slpidlib/PID Controller  Controller=PID  Form=Parallel  TimeDomain=Continuous-time  UseExternalTs=off  SampleTime=0.01  IntegratorMethod=Forward Euler  FilterMethod=Forward Euler  ControllerParametersSource=internal  P=2.50374683332827e-05  I=0.022215359014968  UseKiTs=off  D=0  UseExternalDerivativeSource=off  N=100  UseFilter=on  TunerSelectOption=Transfer Function Based (PID Tuner App)  InitialConditionSource=internal  InitialConditionForIntegrator=0  InitialConditionForFilter=0  DifferentiatorICPrevScaledInput=0  ExternalReset=none  TrackingMode=off  Kt=1  LimitOutput=off  SatLimitsSource=internal  UpperSaturationLimit=inf  LowerSaturationLimit=-inf  LinearizeAsGain=on  AntiWindupMode=none  Kb=1  LimitIntegrator=off  UpperIntegratorSaturationLimit=inf  LowerIntegratorSaturationLimit=-inf  POutMin=[]  POutMax=[]  IOutMin=[]  IOutMax=[]  DOutMin=[]  DOutMax=[]  NOutMin=[]  NOutMax=[]  SumOutMin=[]  SumOutMax=[]  SaturationOutMin=[]  SaturationOutMax=[]  PParamMin=[]  PParamMax=[]  IParamMin=[]  IParamMax=[]  DParamMin=[]  DParamMax=[]  NParamMin=[]  NParamMax=[]  KbParamMin=[]  KbParamMax=[]  KtParamMin=[]  KtParamMax=[]  KbOutMin=[]  KbOutMax=[]  KtOutMin=[]  KtOutMax=[]  IntegratorOutMin=[]  IntegratorOutMax=[]  FilterOutMin=[]  FilterOutMax=[]  SumI1OutMin=[]  SumI1OutMax=[]  SumI2OutMin=[]  SumI2OutMax=[]  SumI3OutMin=[]  SumI3OutMax=[]  SumI4OutMin=[]  SumI4OutMax=[]  SumDOutMin=[]  SumDOutMax=[]  DifferentiatorOutMin=[]  DifferentiatorOutMax=[]  FilterDiffOutCoefMin=[]  FilterDiffOutCoefMax=[]  ReciprocalOutMin=[]  ReciprocalOutMax=[]  SumDenOutMin=[]  SumDenOutMax=[]  SumNumOutMin=[]  SumNumOutMax=[]  DivideOutMin=[]  DivideOutMax=[]  UdiffTsProdOutMin=[]  UdiffTsProdOutMax=[]  NTsProdOutMin=[]  NTsProdOutMax=[]  UintegralTsProdOutMin=[]  UintegralTsProdOutMax=[]  UngainTsProdOutMin=[]  UngainTsProdOutMax=[]  ClampingZeroOutDataTypeStr=Inherit: Inherit via back propagation  ClampingZeroOutMin=[]  ClampingZeroOutMax=[]  FilterDenConstantOutDataTypeStr=Inherit: Inherit via back propagation  FilterDenConstantOutMin=[]  FilterDenConstantOutMax=[]  PCopyOutDataTypeStr=Inherit: Inherit via back propagation  PCopyOutMin=[]  PCopyOutMax=[]  NCopyOutDataTypeStr=Inherit: Inherit via back propagation  NCopyOutMin=[]  NCopyOutMax=[]  IntegratorContinuousStateAttributes=''  IntegratorStateMustResolveToSignalObject=off  IntegratorRTWStateStorageClass=Auto  FilterContinuousStateAttributes=''  FilterStateMustResolveToSignalObject=off  FilterRTWStateStorageClass=Auto  ParallelPVariant=InternalParameters  IdealPVariant=Disabled  IVariant=InternalParameters  DVariant=InternalParameters  IntegratorVariant=Continuous  SatVariant=Disabled  AWVariant=Passthrough  PCopyVariant=Disabled  TRVariant=Disabled  FdbkBlocksVariant=Forward  IdealPFdbkVariant=Disabled  SatFdbkVariant=Disabled  DerivativeFilterVariant=ContFilter  NVariant=InternalParameters  NCopyVariant=Disabled  FilterICVariant=InternalICsFilter  IntegratorICVariant=InternalICs  ExternalResetVariant=Disabled  TRSumVariant=Passthrough  SumFdbkVariant=Disabled  SumVariant=Sum_PID  TsampFilterVariant=InternalTs  TsampNgainVariant=Passthrough  TsampIntegralVariant=Disabled_SignalSpec  ExternalSaturationOutDataTypeStr=Inherit: Same as second input  DerivativeSourceVariant=ErrorSignal
  V limit : Saturate  UpperLimit=20  LowerLimit=-20
  w limit : Saturate  UpperLimit=RW_wmax  LowerLimit=-RW_wmax
  RW1_H : Outport  VectorParamsAs1DForOutWhenUnconnected=off
  RW1_w : Outport  Port=2  VectorParamsAs1DForOutWhenUnconnected=off
  RW1_Hdot : Outport  Port=3  VectorParamsAs1DForOutWhenUnconnected=off
  wires:
  Torque Controller/1 -> V limit/1
  RW - DC Motor Model/3(RW_Hrw_dot) -> RW1_Hdot/1, Sum1/2
  Mux/1 -> "Scope Desired and controlled RW-angular speed "/1
  V limit/1 -> Gain1/1
  Gain1/1 -> RW - DC Motor Model/1(V-rw)  "V-rw"
  RW - DC Motor Model/2(RW_w) -> RW1_w/1, Sum2/2, Mux/2
  Sum1/1 -> Torque Controller/1
  RW - DC Motor Model/1(RW_Hrw) -> RW1_H/1
  Speed Controller1/1 -> w limit/1
  w limit/1 -> Sum1/1
  Sum2/1 -> Speed Controller1/1  "M-error"
  Integrator/1 -> Gain2/1
  RW1_Hdot_des/1 -> Integrator/1
  Gain2/1 -> Mux/1, Sum2/1

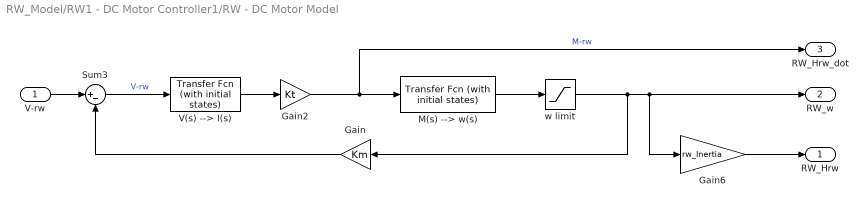
== system RW_Model/RW1 - DC Motor Controller1/RW - DC Motor Model ==
  V-rw : Inport
  Gain : Gain  Gain=Km
  Gain2 : Gain  Gain=Kt
  Gain6 : Gain  Gain=rw_Inertia
  M(s) --> w(s) : simulink_extras/Additional Linear/Transfer Fcn (with initial states)  N=[1]  D=[rw_Inertia b]  X0=0
  Sum3 : Sum  Inputs=|+-
  V(s) --> I(s) : simulink_extras/Additional Linear/Transfer Fcn (with initial states)  N=1  D=[L R]  X0=0
  w limit : Saturate  UpperLimit=RW_wmax  LowerLimit=-RW_wmax
  RW_Hrw : Outport  VectorParamsAs1DForOutWhenUnconnected=off
  RW_w : Outport  Port=2  VectorParamsAs1DForOutWhenUnconnected=off
  RW_Hrw_dot : Outport  Port=3  VectorParamsAs1DForOutWhenUnconnected=off
  wires:
  V-rw/1 -> Sum3/1
  Gain2/1 -> M(s) --> w(s)/1, RW_Hrw_dot/1  "M-rw"
  Gain6/1 -> RW_Hrw/1
  Gain/1 -> Sum3/2
  M(s) --> w(s)/1 -> w limit/1
  Sum3/1 -> V(s) --> I(s)/1  "V-rw"
  V(s) --> I(s)/1 -> Gain2/1
  w limit/1 -> RW_w/1, Gain6/1, Gain/1

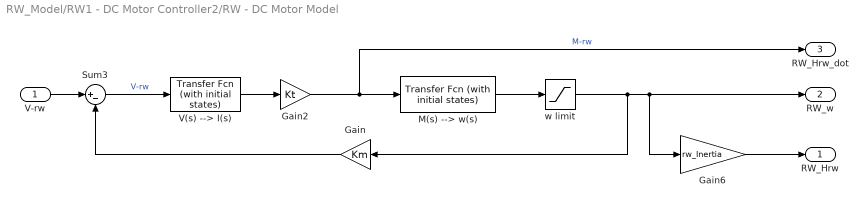
== system RW_Model/RW1 - DC Motor Controller2/RW - DC Motor Model ==
  V-rw : Inport
  Gain : Gain  Gain=Km
  Gain2 : Gain  Gain=Kt
  Gain6 : Gain  Gain=rw_Inertia
  M(s) --> w(s) : simulink_extras/Additional Linear/Transfer Fcn (with initial states)  N=[1]  D=[rw_Inertia b]  X0=0
  Sum3 : Sum  Inputs=|+-
  V(s) --> I(s) : simulink_extras/Additional Linear/Transfer Fcn (with initial states)  N=1  D=[L R]  X0=0
  w limit : Saturate  UpperLimit=RW_wmax  LowerLimit=-RW_wmax
  RW_Hrw : Outport  VectorParamsAs1DForOutWhenUnconnected=off
  RW_w : Outport  Port=2  VectorParamsAs1DForOutWhenUnconnected=off
  RW_Hrw_dot : Outport  Port=3  VectorParamsAs1DForOutWhenUnconnected=off
  wires:
  V-rw/1 -> Sum3/1
  Gain2/1 -> M(s) --> w(s)/1, RW_Hrw_dot/1  "M-rw"
  Gain6/1 -> RW_Hrw/1
  Gain/1 -> Sum3/2
  M(s) --> w(s)/1 -> w limit/1
  Sum3/1 -> V(s) --> I(s)/1  "V-rw"
  V(s) --> I(s)/1 -> Gain2/1
  w limit/1 -> RW_w/1, Gain6/1, Gain/1

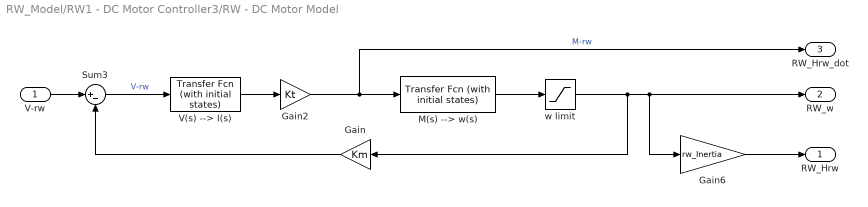
== system RW_Model/RW1 - DC Motor Controller3/RW - DC Motor Model ==
  V-rw : Inport
  Gain : Gain  Gain=Km
  Gain2 : Gain  Gain=Kt
  Gain6 : Gain  Gain=rw_Inertia
  M(s) --> w(s) : simulink_extras/Additional Linear/Transfer Fcn (with initial states)  N=[1]  D=[rw_Inertia b]  X0=0
  Sum3 : Sum  Inputs=|+-
  V(s) --> I(s) : simulink_extras/Additional Linear/Transfer Fcn (with initial states)  N=1  D=[L R]  X0=0
  w limit : Saturate  UpperLimit=RW_wmax  LowerLimit=-RW_wmax
  RW_Hrw : Outport  VectorParamsAs1DForOutWhenUnconnected=off
  RW_w : Outport  Port=2  VectorParamsAs1DForOutWhenUnconnected=off
  RW_Hrw_dot : Outport  Port=3  VectorParamsAs1DForOutWhenUnconnected=off
  wires:
  V-rw/1 -> Sum3/1
  Gain2/1 -> M(s) --> w(s)/1, RW_Hrw_dot/1  "M-rw"
  Gain6/1 -> RW_Hrw/1
  Gain/1 -> Sum3/2
  M(s) --> w(s)/1 -> w limit/1
  Sum3/1 -> V(s) --> I(s)/1  "V-rw"
  V(s) --> I(s)/1 -> Gain2/1
  w limit/1 -> RW_w/1, Gain6/1, Gain/1

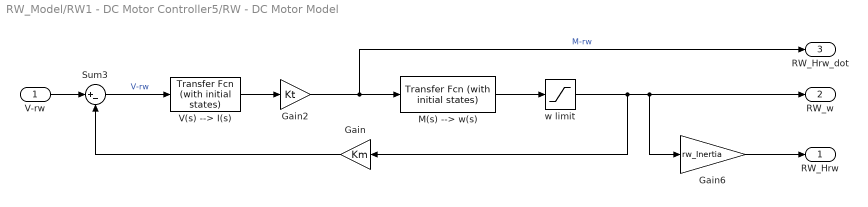
== system RW_Model/RW1 - DC Motor Controller5/RW - DC Motor Model ==
  V-rw : Inport
  Gain : Gain  Gain=Km
  Gain2 : Gain  Gain=Kt
  Gain6 : Gain  Gain=rw_Inertia
  M(s) --> w(s) : simulink_extras/Additional Linear/Transfer Fcn (with initial states)  N=[1]  D=[rw_Inertia b]  X0=0
  Sum3 : Sum  Inputs=|+-
  V(s) --> I(s) : simulink_extras/Additional Linear/Transfer Fcn (with initial states)  N=1  D=[L R]  X0=0
  w limit : Saturate  UpperLimit=RW_wmax  LowerLimit=-RW_wmax
  RW_Hrw : Outport  VectorParamsAs1DForOutWhenUnconnected=off
  RW_w : Outport  Port=2  VectorParamsAs1DForOutWhenUnconnected=off
  RW_Hrw_dot : Outport  Port=3  VectorParamsAs1DForOutWhenUnconnected=off
  wires:
  V-rw/1 -> Sum3/1
  Gain2/1 -> M(s) --> w(s)/1, RW_Hrw_dot/1  "M-rw"
  Gain6/1 -> RW_Hrw/1
  Gain/1 -> Sum3/2
  M(s) --> w(s)/1 -> w limit/1
  Sum3/1 -> V(s) --> I(s)/1  "V-rw"
  V(s) --> I(s)/1 -> Gain2/1
  w limit/1 -> RW_w/1, Gain6/1, Gain/1

== matlab function RW_Model/pseudo inverse ==
  data: u input; y output
function y = pseudoinv(u)

y = pinv(u);

== matlab function RW_Model/Reaction Wheel Model ==
  data: rw_SensorToBody input; Hrw_dot_des output; inv_rwSensorToBody input; Mc input; w_IB_B input; wRw input
function Hrw_dot_des = rwModel(rw_SensorToBody,inv_rwSensorToBody,Mc,w_IB_B,wRw)
% The desired torque is calculated for each reaction wheel 

% The required momentum input
% wRw               (4x1) matrix
% rwInertia_matrix  (4x4) matrix
% rw_SensorToBody   (3x4) matrix
rwInertia = 5e-4; % RW moment of inertia (kg-m2)
rwInertia_matrix = eye(4,4)* rwInertia;
Hrw = rwInertia_matrix * wRw; 

% Hrw_B     (3x1) matrix
% Hrw_B_dot (3x1) matrix
% From Actuator Frame to Satellite Body Frame
Hrw_B = rw_SensorToBody * Hrw ;

% Desired reaction wheel torque in Body Frame
Hrw_B_dot = -Mc - cross(w_IB_B,Hrw_B) ;

% Desired reaction wheel torque in Actuator Frame
Hrw_dot_des = inv_rwSensorToBody * Hrw_B_dot ; 

end
